simulink model "waypoint_generation_ptCloud_200722_mapdata_filtering_6m_1"  (R2020a)
settings: Solver=ode4  StartTime=0.0  StopTime=300  FixedStep=0.01  RelTol=1e-3  EnableMultiTasking=on
InitFcn:
  | detector = load('ptOPDetector.mat');
  | OPdetector = detector.OPdetector;
undefined symbols (not defined in the file): g, Kd_p, Kd_q, Kd_r, Kd_vx, Kd_vy, Kd_vz, Kff_r, Kff_vx, Kff_vy, Kff_vz, Ki_p, Ki_q, Ki_r, Ki_vx, Ki_vy, Ki_vz, Kp_p, Kp_phi, Kp_psi, Kp_q, Kp_r, Kp_theta, Kp_vx, Kp_vy, Kp_vz, M, pointCloud_center, sigma_motor, w_h
libraries: visiontextngfix x4, sharedtransform x1, shared6dof x1, simulink_extras x1
(part 3 of 3)

== matlab function waypoint_generation_ptCloud_200722_mapdata_filtering_6m_1/Path Guidance/MATLAB Function1 ==
  data: w input; yaw output; x input; y input; z input
function yaw = quat2yaw(w,x,y,z)

euler_angle = quat2eul([w x y z],'ZYX');
yaw = euler_angle(1);
end
